simulink model "Pole_placement"  (R2023b)
settings: Solver=VariableStepAuto  StartTime=0.0  StopTime=100  RelTol=1e-3
values from neighbouring files (symbols this model uses):
  A = double(A)    [consistent.m]    (also in dyn_model_mark.m)
  B = double(B)    [consistent.m]    (also in dyn_model_mark.m)
  K = place(A,B,P)    [consistent.m]    (also in dyn_model_mark.m)
  ss_gain = 1/dcgain(cl_lq)    [consistent.m]    (also in dyn_model_mark.m = 1/dcgain(syst_cl))
  x1_bar = 0    [consistent.m]    (also in dyn_model_mark.m)
libraries: simulink_extras x2
settings Model: Creator=Mark  LastModifiedBy=Mark

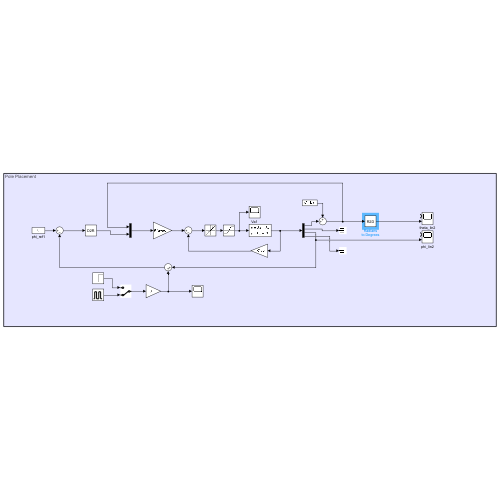
[thumbnail: Simulink's stored preview of the top-level diagram]
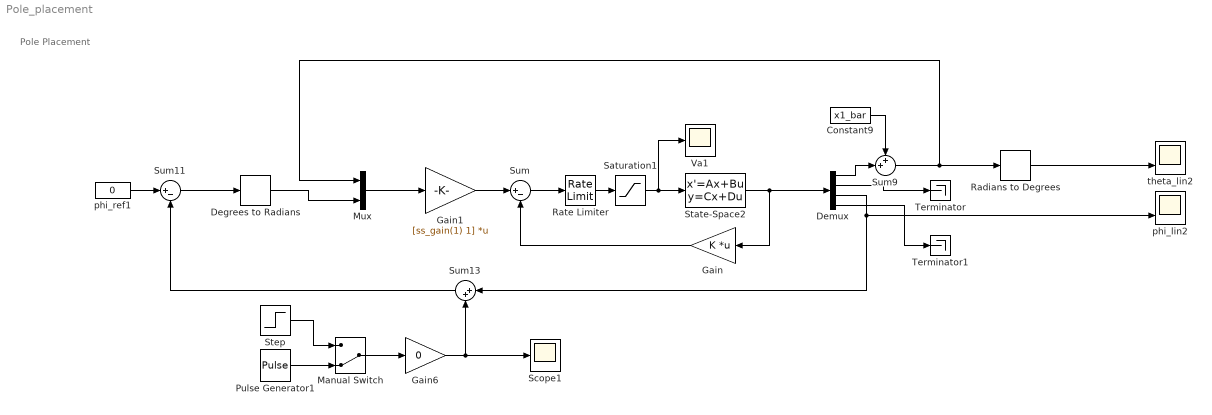
== system Pole_placement ==
  note: Pole Placement
  Constant9 : Constant  Value=x1_bar
  Degrees to Radians : simulink_extras/Transformations/Degrees to Radians
  Demux : Demux
  Gain : Gain  Gain=K  Multiplication=Matrix(K*u) (u vector)
  Gain1 : Gain  Gain=[ss_gain(1) 1]  Multiplication=Matrix(K*u) (u vector)
  Gain6 : Gain  Gain=0
  Manual Switch : ManualSwitch  CurrentSetting=0
  Mux : Mux  Inputs=2
  Pulse Generator1 : DiscretePulseGenerator  PulseType=Time based  Period=10000  PulseWidth=0.005  PhaseDelay=30
  Radians to Degrees : simulink_extras/Transformations/Radians to Degrees
  Rate Limiter : RateLimiter  RisingSlewLimit=inf  FallingSlewLimit=-inf  SampleTimeMode=inherited
  Saturation1 : Saturate  UpperLimit=10  LowerLimit=-10
  Scope1 : Scope
  State-Space2 : StateSpace  A=A  B=B  C=[1 0 0 0; 0 1 0 0; 0 0 1 0; 0 0 0 1]  D=[0 0 0 0]'  InitialCondition=[0 0 90*pi/180 0]
  Step : Step  Time=30  SampleTime=0
  Sum : Sum  Inputs=|+-
  Sum11 : Sum  Inputs=|+-
  Sum13 : Sum  Inputs=|++
  Sum9 : Sum  Inputs=++|
  Terminator : Terminator
  Terminator1 : Terminator
  Va1 : Scope
  phi_lin2 : Scope  NumInputPorts=2
  phi_ref1 : Constant  Value=0
  theta_lin2 : Scope  NumInputPorts=2
  wires:
  phi_ref1/1 -> Sum11/1
  Degrees to Radians/1 -> Mux/2
  Sum9/1 -> Radians to Degrees/1, Mux/1
  Pulse Generator1/1 -> Manual Switch/2
  Sum11/1 -> Degrees to Radians/1
  Gain6/1 -> Scope1/1, Sum13/2
  Constant9/1 -> Sum9/1
  Step/1 -> Manual Switch/1
  Radians to Degrees/1 -> theta_lin2/2
  Sum13/1 -> Sum11/2
  Manual Switch/1 -> Gain6/1
  State-Space2/1 -> Gain/1, Demux/1
  Gain/1 -> Sum/2
  Saturation1/1 -> Va1/1, State-Space2/1
  Demux/3 -> phi_lin2/2, Sum13/1
  Demux/1 -> Sum9/2
  Gain1/1 -> Sum/1
  Demux/2 -> Terminator/1
  Demux/4 -> Terminator1/1
  Mux/1 -> Gain1/1
  Sum/1 -> Rate Limiter/1
  Rate Limiter/1 -> Saturation1/1
